simulink model "fahrbahn"  (Simulink 3.00)
settings: Solver=ode4  StartTime=0.0  StopTime=10.0  FixedStep=0.01  RelTol=1e-3
settings Model: LastModifiedBy=student

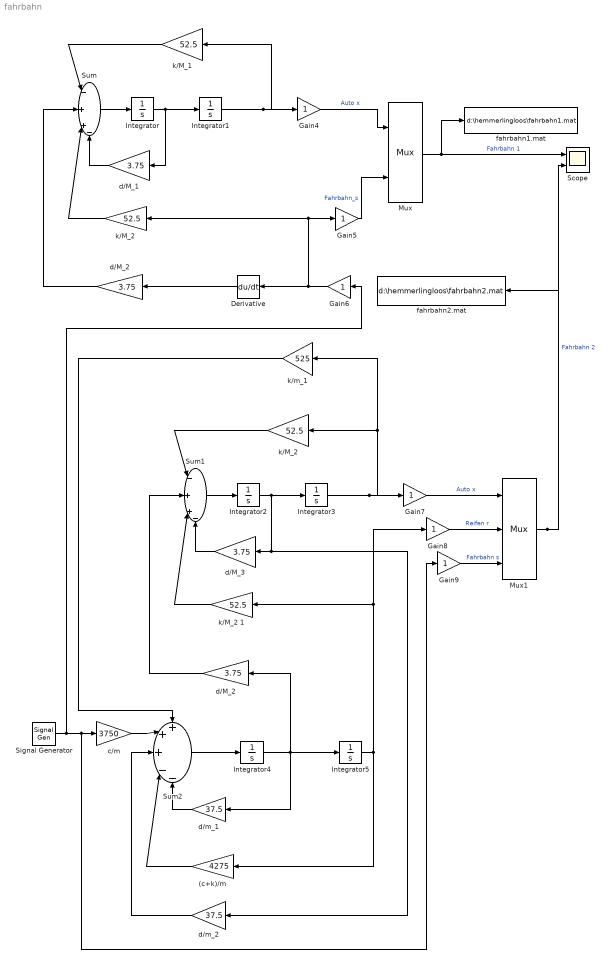
== system fahrbahn ==
  (c+k)/m : Gain  Orientation=left  Gain=4275  SaturateOnIntegerOverflow=on
  Derivative : Derivative  Orientation=left
  Gain{4..5,7..9} (5 alike) : Gain  Gain=1  SaturateOnIntegerOverflow=on
  Gain6 : Gain  Orientation=left  Gain=1  SaturateOnIntegerOverflow=on
  Integrator{,1..5} (6 alike) : Integrator  ExternalReset=none  InitialConditionSource=internal  InitialCondition=0  LimitOutput=off  UpperSaturationLimit=inf  LowerSaturationLimit=-inf  ShowSaturationPort=off  ShowStatePort=off  AbsoluteTolerance=auto
  Mux : Mux  Inputs=2
      settings: DisplayOption=signals
  Mux1 : Mux  Inputs=3
      settings: DisplayOption=signals
  Scope : Scope  NumInputPorts=2
      settings: TimeRange=1  YMin=0~-5  YMax=1~5  SaveToWorkspace=off  SaveName=ScopeData
  Signal Generator : SignalGenerator  WaveForm=sine  Amplitude=0.1  Frequency=10  Units=Hertz
  Sum : Sum  Inputs=|-++-  SaturateOnIntegerOverflow=on
  Sum1 : Sum  Inputs=|-++-  SaturateOnIntegerOverflow=on
  Sum2 : Sum  Inputs=+++--  SaturateOnIntegerOverflow=on
  c/m : Gain  Gain=3750  SaturateOnIntegerOverflow=on
  d/M_1 : Gain  Orientation=left  Gain=3.75  SaturateOnIntegerOverflow=on
  d/M_2 : Gain  Orientation=left  Gain=3.75  SaturateOnIntegerOverflow=on
  "d/M_2 " : Gain  Orientation=left  Gain=3.75  SaturateOnIntegerOverflow=on
  d/M_3 : Gain  Orientation=left  Gain=3.75  SaturateOnIntegerOverflow=on
  d/m_1 : Gain  Orientation=left  Gain=37.5  SaturateOnIntegerOverflow=on
  "d/m_2 " : Gain  Orientation=left  Gain=37.5  SaturateOnIntegerOverflow=on
  fahrbahn1.mat : ToFile  Filename=d:\hemmerlingloos\fahrbahn1.mat  MatrixName=ans  SampleTime=-1
  fahrbahn2.mat : ToFile  Orientation=left  Filename=d:\hemmerlingloos\fahrbahn2.mat  MatrixName=ans  SampleTime=-1
  k/M_1 : Gain  Orientation=left  Gain=52.5  SaturateOnIntegerOverflow=on
  k/M_2 : Gain  Orientation=left  Gain=52.5  SaturateOnIntegerOverflow=on
  "k/M_2 " : Gain  Orientation=left  Gain=52.5  SaturateOnIntegerOverflow=on
  k/M_2 1 : Gain  Orientation=left  Gain=52.5  SaturateOnIntegerOverflow=on
  k/m_1 : Gain  Orientation=left  Gain=525  SaturateOnIntegerOverflow=on
  wires:
  Derivative/1 -> d/M_2/1
  Integrator/1 -> Integrator1/1, d/M_1/1
  d/M_1/1 -> Sum/4
  "k/M_2 "/1 -> Sum/3
  d/M_2/1 -> Sum/2
  k/M_1/1 -> Sum/1
  Sum/1 -> Integrator/1
  Integrator1/1 -> Gain4/1, k/M_1/1
  Gain4/1 -> Mux/1  "Auto x"
  Gain5/1 -> Mux/2  "Fahrbahn_s"
  Gain6/1 -> Derivative/1, Gain5/1, "k/M_2 "/1
  Integrator2/1 -> Integrator3/1, d/M_3/1, "d/m_2 "/1
  d/M_3/1 -> Sum1/4
  k/M_2 1/1 -> Sum1/3
  "d/M_2 "/1 -> Sum1/2
  k/M_2/1 -> Sum1/1
  Sum1/1 -> Integrator2/1
  Integrator3/1 -> Gain7/1, k/M_2/1, k/m_1/1
  Gain7/1 -> Mux1/1  "Auto x"
  Gain8/1 -> Mux1/2  "Reifen r"
  Sum2/1 -> Integrator4/1
  Integrator4/1 -> Integrator5/1, "d/M_2 "/1, d/m_1/1
  d/m_1/1 -> Sum2/5
  (c+k)/m/1 -> Sum2/4
  "d/m_2 "/1 -> Sum2/3
  c/m/1 -> Sum2/2
  k/m_1/1 -> Sum2/1
  Integrator5/1 -> (c+k)/m/1, Gain8/1, k/M_2 1/1
  Gain9/1 -> Mux1/3  "Fahrbahn s"
  Signal Generator/1 -> c/m/1, Gain9/1, Gain6/1
  Mux/1 -> Scope/1, fahrbahn1.mat/1  "Fahrbahn 1"
  Mux1/1 -> Scope/2, fahrbahn2.mat/1  "Fahrbahn 2"
